simulink model "etimer_capture"  (Simulink 8.1)
settings: Solver=FixedStepDiscrete  StartTime=0.0  StopTime=10.0  FixedStep=0.2  RelTol=1e-3
undefined symbols (not defined in the file or in its folder): A14, B, B13, D, D16, L3, P3, PD10, PD14, PD6, R10, T15
libraries: rappid_564xl_ec_toolbox x7
settings Model: Creator=evarshavskaya  LastModifiedBy=evarshavskaya
settings DataIOCC: ExternalInput=off  InitialState=off  SaveOutput=off  SignalLogging=off  SaveTime=off
settings OptimizationCC: InlineParams=on  OptimizeModelRefInitCode=on  LifeSpan=1
settings DebuggingCC: InheritedTsInSrcMsg=none  SingleTaskRateTransMsg=error  UnconnectedInputMsg=error  UnconnectedOutputMsg=error  UnconnectedLineMsg=error  UnknownTsInhSupMsg=error
settings HardwareCC: ProdLargestAtomicInteger=Long  ProdLargestAtomicFloat=Double  ProdIntDivRoundTo=Zero  ProdEndianess=BigEndian  ProdHWDeviceType=Freescale->32-bit PowerPC
settings RTWCC: SystemTargetFile=rappid564xl.tlc  MakeCommand=rappid_564xl_make_rtw  TemplateMakefile=rappid_564xl_default_tmf  PostCodeGenCommand=rappid_analyzegencode(buildInfo)  Description=RAppID Toolbox MPC564xL Code Generation Target (rappid)  ProcessScript=rappid564xl_make_rtw_hook
settings CodeAppCC: IgnoreCustomStorageClasses=off  CustomSymbolStrType=$N$R$M  InternalIdentifier=Classic
settings STFCustomTargetCC: CodeReplacementLibrary=ANSI_C  ModelReferenceCompliant=off  CombineOutputUpdateFcns=on  SuppressErrorStatus=on  ERTCustomFileBanners=on  SupportContinuousTime=off  SupportNonInlinedSFcns=off  MATLABClassNameForMDSCustomization=Simulink.SoftwareTarget.ERTCustomization  GRTInterface=off  SystemTargetFile=rappid564xl.tlc
settings ERTTargetCC: CodeReplacementLibrary=ANSI_C  MultiwordLength=2048  ModelReferenceCompliant=off  ParMdlRefBuildCompliant=off  CompOptLevelCompliant=off  ConcurrentExecutionCompliant=off  SuppressErrorStatus=on  ERTFirstTimeCompliant=off  ModelStepFunctionPrototypeControlCompliant=off  CPPClassGenCompliant=off  ExtModeMexFile=noextcomm  InlinedParameterPlacement=NonHierarchical  ERTCustomFileTemplate=example_file_process.tlc  ConvertIfToSwitch=off  SuppressUnreachableDefaultCases=off

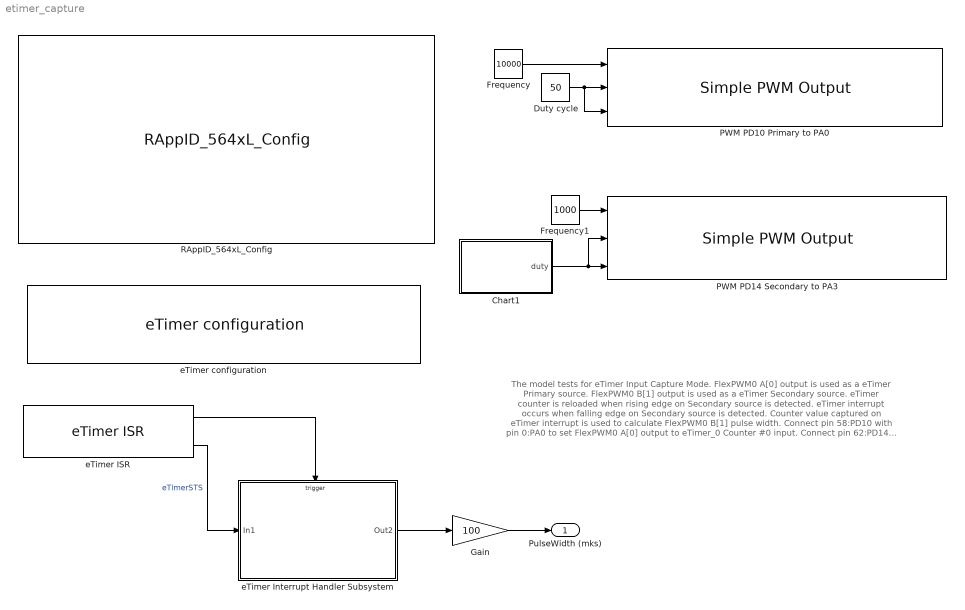
== system etimer_capture ==
  note: The model tests for eTimer Input Capture Mode.
      |
      | FlexPWM0 A[0] output is used as a eTimer Primary source.
      | FlexPWM0 B[1] output is used as a eTimer Secondary source.
      | eTimer counter is reloaded when rising edge on Secondary source is detected.
      | eTimer interrupt occurs when falling edge on Secondary source is detected.
      | Counter value captured on eTimer interrupt is used to calculate FlexPWM0 B[1] pulse width.
      |
      | Connect pin 58:PD10 with pin 0:PA0 to set FlexPWM0 A[0] output to eTimer_0 Counter #0 input.
      | Connect pin 62:PD14 with pin 3:PA3 to set FlexPWM0 B[1] output to eTimer_0 Counter #3 input.
      |
      | Start FreeMaster and open etimer_capture.pmp project to view FlexPWM0 B[1] pulse width
  Chart1 : Stateflow chart  TreatAsAtomicUnit=on
  Duty cycle : Constant  Value=50  OutDataTypeStr=uint32
  Frequency : Constant  Value=10000  OutDataTypeStr=uint32
  Frequency1 : Constant  Value=1000  OutDataTypeStr=uint32
  Gain : Gain  Gain=100  OutDataTypeStr=uint16
  PWM PD10 Primary to PA0 : rappid_564xl_ec_toolbox/MPC564xL/Motor Control Blocks/Simple PWM Output  Priority=1  pwmModule=0  pwmMod=0  SubModule=0  subMod=0  InitFreq=10000  resolution=1 %  resValue=1  InitDutyA=50  InitDutyB=50  align=A B - edge aligned  PhaseShift_A=0  PhaseShift=0  Phase_A=0  Phase_B=0  centered=0  DoubleS=off  doubleSw=off  debugSw=off  debug_mode=0  pin_A0="58  : PD10 : [ 76 ] : [ T15 ]"  pin_B0=None  pin_X0=None  pin_A1=None  pin_B1=None  pin_X1=None  pin_A2=None  pin_B2=None  pin_X2=None  pin_A3=None  pin_B3=None  pin_X3=None  pin1_A0=None  pin1_B0=None  pin1_X0=None  pin1_A1=None  pin1_B1=None  pin1_X1=None  pin1_A2=None  pin1_B2=None  pin1_X2=None  pin1_A3=None  pin1_B3=None  pin1_X3=None  pcrNumA=58  pcrNumB=255  pcrNumX=255  polA=off  polB=off  polX=off  octrl=0  syncFrom0=off  masterSync=0  outVal0=off  outVal1=off  outVal2=off  outVal3=off  outVal4=off  outVal5=off  outTrig=0
  PWM PD14 Secondary to PA3 : rappid_564xl_ec_toolbox/MPC564xL/Motor Control Blocks/Simple PWM Output  Priority=1  pwmModule=0  pwmMod=0  SubModule=1  subMod=1  InitFreq=1000  resolution=1 %  resValue=1  InitDutyA=70  InitDutyB=70  align=A B - edge aligned  PhaseShift_A=0  PhaseShift=0  Phase_A=0  Phase_B=0  centered=0  DoubleS=off  doubleSw=off  debugSw=off  debug_mode=0  pin_A0="58  : PD10 : [ 76 ] : [ T15 ]"  pin_B0=None  pin_X0=None  pin_A1=None  pin_B1="62  : PD14 : [ 105 ] : [ D16 ]"  pin_X1=None  pin_A2=None  pin_B2=None  pin_X2=None  pin_A3=None  pin_B3=None  pin_X3=None  pin1_A0=None  pin1_B0=None  pin1_X0=None  pin1_A1=None  pin1_B1=None  pin1_X1=None  pin1_A2=None  pin1_B2=None  pin1_X2=None  pin1_A3=None  pin1_B3=None  pin1_X3=None  pcrNumA=255  pcrNumB=62  pcrNumX=255  polA=off  polB=off  polX=off  octrl=0  syncFrom0=off  masterSync=0  outVal0=off  outVal1=off  outVal2=off  outVal3=off  outVal4=off  outVal5=off  outTrig=0
  RAppID_564xL_Config : rappid_564xl_ec_toolbox/MPC564xL/RAppID_564xL_Config  SystemClock=120  XTAL=40  MC_clock_60=12  MC_clock_80=16  MC_clock_120=10  SWG_clock_60=20  SWG_clock_80=13.334  SWG_clock_120=20  Compiler=CodeWarrior  MemTarget=RAM  Part=MPC5643L  Package=144 LQFP  global_int_priority=10  base_tick_priority=14  sys_task_supress=off  exception_handlers=off  stored_mdl_name=etimer_capture  freemaster_interface=Oops  freemaster_rx_pin="LINFlex_0 Rx Pin 116 : \"PB[3]\""  freemaster_tx_pin="LINFlex_0 Tx Pin 114 : \"PB[2]\""  freemaster_interface_1=Serial 0  freemaster_enable=on  freemaster_rate=57600  freemaster_tx0_pin=18 : B[2] : 114 : A14  freemaster_rx0_pin=19 : B[3] : 116 : B13  freemaster_tx1_pin=57 : D[9] : 26 : L3  freemaster_rx1_pin=29 : B[13] : 60 : R10  freemaster_can_channel=1CH  freemater_can_speed=500K  freemaster_can_msgig=0x7AA  ccp_interface=None  ccp_enable=off  ccp_can_channel=CH1 (MB 0 - 1)  ccp_can_speed=500K  ccp_can_cro_id=256  ccp_can_dto_id=257  ccp_dev_id=RappID  ccp_dev_addr=0  ccp_odt=3  ccp_daq=3  pil_enable=off  pil_bam=on  comport=1  pil_rate=57600  bam_password_def=on  bam_password=0xFEEDFACECAFEBEEF  bam_sa_cs=off  bam_start_address=0x0  bam_code_size=0x7000  cons_dspi=on  cons_can=on  cons_adc=on  cons_pwm=on  cons_ctu=on  cons_swg=on  cons_eTimer=on  cons_fm=on
  eTimer ISR : rappid_564xl_ec_toolbox/MPC564xL/Motor Control Blocks/eTimer ISR  SubModule=0  Timerchan=1  subMod=0  channel=1  isrPriority=12  isrPrio=12
  eTimer Interrupt Handler Subsystem : Subsystem  TreatAsAtomicUnit=on
      settings: RTWSystemCode=Nonreusable function
  eTimer configuration : rappid_564xl_ec_toolbox/MPC564xL/Motor Control Blocks/eTimer configuration  SubModule=0  TimerChan=1  subMod=0  channel=1  CountMode=001 - Count rising edges of primary source  CNTMODE=1  CountOnce=0 - Count repeatedly  ONCE=0  CountLength=0 - Continue counting to roll over  LENGTH=0  CountDirection=0 - Count up  DIR=0  OutputEnable=1 - Output signal is driven to the external pin  OEN=1  CoChanInit=00 - Other channels cannot force re-initialization of this channel  COINIT=0  StopAction=0 - Output enable is unaffected by stop mode  STPEN=0  ReloadOnCapt=01 - Reload the counter on a capture 1 event  ROC=1  PrimarySource=00000 - Counter #0 input pin  PRISRC=0  PrimSrcPol=0 - True polarity  PIPS=0  SecondarySource=00011 - Counter #3 input pin  SECSRC=3  SecSrcPol=0 - True polarity  SIPS=0  FILT_CNT=0  FILT_PER=0  FILT=0  OutputMode=0000 - Software controlled  OUTMODE=0  OutputPol=0 - True polarity  OPS=0  MasterMode=0 - Disable broadcast of this channel output  MSTR=0  ForcedOutVal=0  VAL=0  CoForce=0 - Other channels cannot force this channel output  COFRC=0  CompLoad1=000 - COMP1 is never preload  CLC1=0  CompLoad2=000 - COMP2 is never preload  CLC2=0  CompareMode="00 - COMP1 and COMP2  are used when the counter is counting up"  CMPMODE=0  CaptMode1=10 - Capture rising edges  CPT1MODE=2  CaptMode2=01 - Capture falling edges  CPT2MODE=1  OneShCaptMode=0 - Free running mode is selected  ONESHOT=0  CaptFIFO=0  CFWM=0  CNTRinit=0  COMP1init=0  COMP2init=0  mod0ch0pin="0   : PA0  : [ 73 ] : [ T14 ]  input/output"  mod0ch1pin=None  mod0ch2pin=None  mod0ch3pin="3   : PA3  : [ 92 ] : [ K17 ]  input/output"  mod0ch4pin=None  mod0ch5pin=None  mod1ch0pin=None  mod1ch1pin=None  mod1ch2pin=None  mod1ch3pin=None  mod1ch4pin=None  mod1ch5pin=None  mod2ch0pin=None  mod2ch1pin=None  mod2ch2pin=None  mod2ch3pin=None  mod2ch4pin=None  mod2ch5pin=None  pcrNum0=0  pcrNum1=255  pcrNum2=255  pcrNum3=3  pcrNum4=255  pcrNum5=255  TCFIE=off  TCF1IE=off  TCF2IE=off  TOFIE=off  IELFIE=off  IEHFIE=off  ICF1IE=off  ICF2IE=on  INTDMA=128
  PulseWidth (mks) : Outport
  wires:
  eTimer ISR/1 -> eTimer Interrupt Handler Subsystem/Trigger
  eTimer ISR/2 -> eTimer Interrupt Handler Subsystem/1(In1)  "eTimerSTS"
  Frequency/1 -> PWM PD10 Primary to PA0/1
  Frequency1/1 -> PWM PD14 Secondary to PA3/1
  Duty cycle/1 -> PWM PD10 Primary to PA0/2, PWM PD10 Primary to PA0/3
  eTimer Interrupt Handler Subsystem/1(Out2) -> Gain/1
  Chart1/1(duty) -> PWM PD14 Secondary to PA3/3, PWM PD14 Secondary to PA3/2
  Gain/1 -> PulseWidth (mks)/1

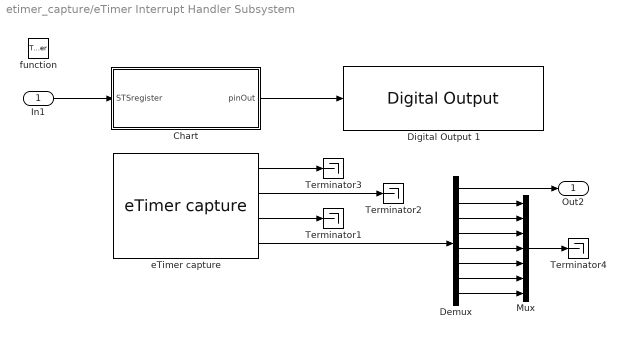
== system etimer_capture/eTimer Interrupt Handler Subsystem ==
  In1 : Inport
  function : TriggerPort  TriggerType=function-call
  Chart : Stateflow chart  TreatAsAtomicUnit=on
  Demux : Demux  Outputs=8
  Digital Output 1 : rappid_564xl_ec_toolbox/MPC564xL/General Purpose Blocks/Digital Output   gpio_outputs="54  : PD6  : [ 34 ] : [ P3 ]"  pinNum=[ 34 ]  pcrNum=54
  Mux : Mux  Inputs=7
  Terminator{1..4} (4 alike) : Terminator
  eTimer capture : rappid_564xl_ec_toolbox/MPC564xL/Motor Control Blocks/eTimer capture  SubModule=0  Timerchan=1  subMod=0  channel=1
  Out2 : Outport
  wires:
  eTimer capture/1 -> Terminator3/1
  eTimer capture/2 -> Terminator2/1
  In1/1 -> Chart/1(STSregister)
  Chart/1(pinOut) -> Digital Output 1/1
  eTimer capture/3 -> Terminator1/1
  eTimer capture/4 -> Demux/1
  Demux/8 -> Mux/7
  Demux/7 -> Mux/6
  Demux/6 -> Mux/5
  Demux/5 -> Mux/4
  Demux/4 -> Mux/3
  Demux/3 -> Mux/2
  Demux/2 -> Mux/1
  Mux/1 -> Terminator4/1
  Demux/1 -> Out2/1

== stateflow chart Chart1 ==
  settings: executeAtInitialization=1
  state A
    du:
    duty=cntr*10;
    cntr=cntr+1;
  state A1
    du:
    duty=cntr*10;
    cntr=cntr-1;
  (default) -> A : {cntr=1;}
  A1 -> A : [cntr < 2]
  A -> A1 : [cntr > 8]
  data: cntr local uint32 [0..1000] =0; duty output uint32 [0..100]

== stateflow chart eTimer Interrupt Handler Subsystem/Chart ==
  state A
    du:
    compare = STSregister & 2;
    en:
    compare = STSregister & 2;
    pinOut = 1;
  state A1
    du:
    compare = STSregister & 2;
    en:
    compare = STSregister & 2;
    pinOut = 0;
  (default) -> A
  A -> A1 : [compare == 0]
  A1 -> A : [compare != 0]
  data: compare local int16 [0..2]; pinOut output boolean [0..1]; STSregister input uint16 [0..65535]
